simulink model "rpi_bird_eye_view_1"  (R2016a)
settings: Solver=FixedStepAuto  StartTime=0.0  StopTime=inf  RelTol=1e-3
libraries: visiongeotforms x2, embdlinuxlib x2
settings Model: SimulationMode=external  Creator=Yewly  LastModifiedBy=Yewly
settings SolverCC: PositivePriorityOrder=on
settings OptimizationCC: OptimizeModelRefInitCode=on  LifeSpan=1  MaxStackSize=64
settings HardwareCC: ProdBitPerPointer=32  ProdLargestAtomicInteger=Long  ProdLargestAtomicFloat=Double  ProdWordSize=32  ProdHWDeviceType=ARM Compatible->ARM Cortex
settings RTWCC: SystemTargetFile=ert.tlc  HardwareBoard=Raspberry Pi  TemplateMakefile=ert_default_tmf  GenerateReport=on  Toolchain=GNU GCC Raspberry Pi  IncludeHyperlinkInReport=on  LaunchReport=on  GenerateTraceInfo=on  GenerateTraceReport=on  GenerateTraceReportSl=on  GenerateTraceReportSf=on  GenerateTraceReportEml=on
settings CodeAppCC: ForceParamTrailComments=on  IgnoreCustomStorageClasses=off  OperatorAnnotations=on  SimulinkDataObjDesc=on  SFDataObjDesc=on  MATLABFcnDesc=on  InsertBlockDesc=on  MATLABSourceComments=on
settings ERTTargetCC: SupportVariableSizeSignals=on

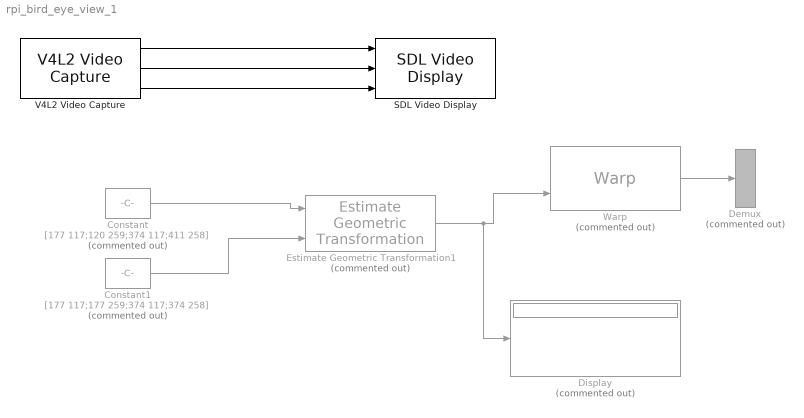
== system rpi_bird_eye_view_1 ==
  Constant : Constant  Commented=on  Value=[177 117;120 259;374 117;411 258]
  Constant1 : Constant  Commented=on  Value=[177 117;177 259;374 117;374 258]
  Demux : Demux  Commented=on  Outputs=3
  Display : Display  Commented=on
  Estimate Geometric Transformation1 : visiongeotforms/Estimate Geometric Transformation  Commented=on  tformType=Projective  isRandomSampling=on  algMethod=Random Sample Consensus (RANSAC)  numMethod=Specified value  isStopSampling=off  percentStop=75  distanceAlg=2.5  distanceGeo=2.5  sampleNum=500  maxSampleNum=1000  desiredConfidence=99  isRefineTForm=off  isOutputInlier=off  outDT4IntInput=Obsolete10a  outDT4IntInputActive=Single  isVarSizeAllowed=on  isReleaseMode=on
  SDL Video Display : embdlinuxlib/SDL Video Display  pixelFormat=RGB  pixelOrder=Planar  rowMajor=on  blockPlatform=Raspberry Pi
  V4L2 Video Capture : embdlinuxlib/V4L2 Video Capture  m_devName='/dev/video0'  roi=[0, 0, 640, 480]  imSizeSelection=320x240  imSize=[640, 480]  pixelFormat=RGB  pixelOrder=Planar  sampleTime=1/10  simOutput=Colorbars  blockPlatform=Raspberry Pi
  Warp : visiongeotforms/Warp  Commented=on  TransformMatrixSource=Input port  TransformMatrix=eye( 3 )  InterpolationMethod=Bilinear  BackgroundFillValue=0  OutputImagePositionSource=Same as input image  OutputImagePosition=[ 1, 1, 512, 512 ]  ROIInputPort=off  ROIValidityOutputPort=off  SimulateUsing=Interpreted execution
  wires:
  Estimate Geometric Transformation1/1 -> Display/1, Warp/2
  Constant/1 -> Estimate Geometric Transformation1/1
  Constant1/1 -> Estimate Geometric Transformation1/2
  V4L2 Video Capture/1 -> SDL Video Display/1
  V4L2 Video Capture/2 -> SDL Video Display/2
  V4L2 Video Capture/3 -> SDL Video Display/3
  Warp/1 -> Demux/1
